simulink model "ControladoresPIDv5"  (R2020a)
settings: Solver=ode5  StartTime=0.0  StopTime=20  FixedStep=0.0001  RelTol=1e-3
values from neighbouring files (symbols this model uses):
  Bm = 0.008    [definirParametros.m]    (also in definirParametrosMotorElectroCraftDP300.m; definirParametrosMotorElectroCraftDPP728V120.m = Jm/tm; definirParametrosMotorElectroCraftDPP728V120_Optimizador.m = Jm/tm; definirParametrosMotorElectroCraftDPP728V120_v2.m = Jm/tm)
  dm = 0.3    [definirParametros.m]    (also in definirParametrosMotorElectroCraftDP300.m; definirParametrosMotorElectroCraftDPP728V120.m; definirParametrosMotorElectroCraftDPP728V120_Optimizador.m = 0.550061; definirParametrosMotorElectroCraftDPP728V120_v2.m = 0.550061)
  dmc = 0.5    [definirParametros.m]    (also in definirParametrosMotorElectroCraftDP300.m; definirParametrosMotorElectroCraftDPP728V120.m; definirParametrosMotorElectroCraftDPP728V120_Optimizador.m = 1.06911; definirParametrosMotorElectroCraftDPP728V120_v2.m = 1.06911)
  g = 9.8    [definirParametros.m]    (also in definirParametrosMotorElectroCraftDP300.m; definirParametrosMotorElectroCraftDPP728V120.m; definirParametrosMotorElectroCraftDPP728V120_Optimizador.m; definirParametrosMotorElectroCraftDPP728V120_v2.m)
  Jm = gramsCM2ToKgMeters2(12358.5)    [definirParametrosMotorElectroCraftDPP728V120.m]    (also in definirParametrosMotorElectroCraftDPP728V120_Optimizador.m; definirParametrosMotorElectroCraftDPP728V120_v2.m; definirParametrosMotorElectroCraftDPP728V120_v3.m; definirParametrosMotorElectroCraftRP34M221V90.m = gramsCM2ToKgMeters2(2718.9))
  Kb = 0.6    [definirParametros.m]    (also in definirParametrosMotorElectroCraftDP300.m = VoltagePerKRPMToVoltagePerHertz(12.3); definirParametrosMotorElectroCraftDPP728V120.m = VoltagePerKRPMToVoltagePerRadS(64.9); definirParametrosMotorElectroCraftDPP728V120_Optimizador.m = VoltagePerKRPMToVoltagePerRadS(64.9); definirParametrosMotorElectroCraftDPP728V120_v2.m = VoltagePerKRPMToVoltagePerRadS(64.9))
  Kt = 0.7274    [definirParametros.m]    (also in definirParametrosMotorElectroCraftDP300.m = newtonCMToNewtonM(11.722); definirParametrosMotorElectroCraftDPP728V120.m = newtonCMToNewtonM(62); definirParametrosMotorElectroCraftDPP728V120_Optimizador.m = newtonCMToNewtonM(62); definirParametrosMotorElectroCraftDPP728V120_v2.m = newtonCMToNewtonM(62))
  Lm = 4.3/1000    (= 0.0043)    [definirParametrosMotorElectroCraftDPP728V120.m]    (also in definirParametrosMotorElectroCraftDPP728V120_Optimizador.m; definirParametrosMotorElectroCraftDPP728V120_v2.m; definirParametrosMotorElectroCraftDPP728V120_v3.m; definirParametrosMotorElectroCraftDPP728V60.m = 0.0015)
  Mc = 200    [definirParametros.m]    (also in definirParametrosMotorElectroCraftDP300.m; definirParametrosMotorElectroCraftDPP728V120.m; definirParametrosMotorElectroCraftDPP728V120_Optimizador.m = 144.6; definirParametrosMotorElectroCraftDPP728V120_v2.m = 144.6)
  Mm = 100    [definirParametros.m]    (also in definirParametrosMotorElectroCraftDP300.m; definirParametrosMotorElectroCraftDPP728V120.m; definirParametrosMotorElectroCraftDPP728V120_Optimizador.m = 18.911; definirParametrosMotorElectroCraftDPP728V120_v2.m = 18.911)
  relacionEngranajes = 100.0/1    (= 100)    [definirParametros.m]    (also in definirParametrosMotorElectroCraftDP300.m = 1; definirParametrosMotorElectroCraftDPP728V120.m; definirParametrosMotorElectroCraftDPP728V120_Optimizador.m; definirParametrosMotorElectroCraftDPP728V120_v2.m)
  Rm = 1.55    [definirParametrosMotorElectroCraftDPP728V120.m]    (also in definirParametrosMotorElectroCraftDPP728V120_Optimizador.m; definirParametrosMotorElectroCraftDPP728V120_v2.m; definirParametrosMotorElectroCraftDPP728V120_v3.m; definirParametrosMotorElectroCraftDPP728V60.m = 0.72)
libraries: simulink x13
settings Model: Creator=rghuertaspaiva  LastModifiedBy=rghuertaspaiva

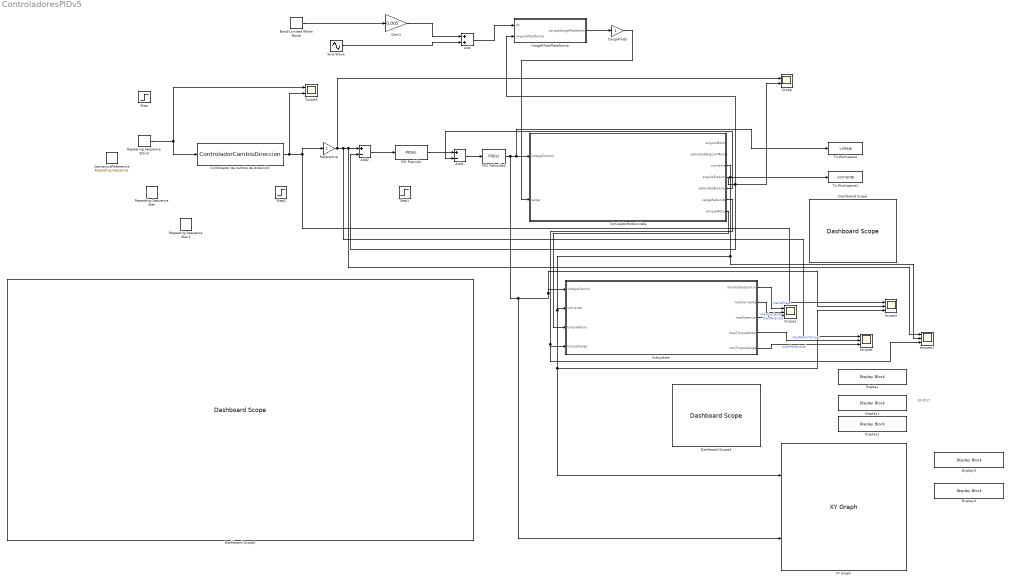
== system ControladoresPIDv5 ==
  note: 18.4917
  Add : Sum
  Add1 : Sum  Inputs=+-
  Add2 : Sum  Inputs=+-
  Band-Limited White Noise : simulink/Sources/Band-Limited White Noise  Cov=[.1]  Ts=0.001  seed=[23341]
  CargaPiloto : Gain
  CargaPilotoPlataforma : Subsystem
  Controlador de cambio de dirección : S-Function  InitFcn=try, set_param(gcb,'FunctionName','ControladorCambioDireccion'), end  FunctionName=ControladorCambioDireccion  SFunctionModules=ControladorCambioDireccion_wrapper  SFunctionDeploymentMode=off  EnableBusSupport=off  mask(S-Function Builder){}
      mask help: Simulink:masks:SFunctionBuilder_MD
      mask init:
      | val = [[.9  0.75 0.75 1 1 .9 .9 1]',[1 1 0.75 0.75 .9 .9 1 .9]'];try , sys = get_param(gcb,'SfunBuilderFcnName');if isempty(sys), sys = get_param(gcb,'FunctionName'); end,catch, sys = get_param(gcb,'FunctionName'); end
      settings: CopyFcn=set_param(gcbh,'LinkStatus','none')  PreSaveFcn=try, set_param(gcb,'FunctionName','ControladorCambioDireccion'), end  OpenFcn=sfunctionwizard(gcbh)
      mask Display: plot(val(:,1),val(:,2)),disp(sys), port_label('input',1,'entrada'), port_label('output',1,'salida')
  Dashboard Scope : DashboardScope
  Dashboard Scope2 : DashboardScope
  Dashboard Scope3 : DashboardScope
  Display{,1..4} (5 alike) : DisplayBlock  LabelPosition=Hide  Format=short  Transparency=1
  Gain1 : Gain  Gain=0.005
  PID Posiciǿn : simulink/Continuous/PID Controller  Controller=PID  Form=Parallel  TimeDomain=Continuous-time  UseExternalTs=off  SampleTime=-1  IntegratorMethod=Forward Euler  FilterMethod=Forward Euler  ControllerParametersSource=internal  P=21  I=0  D=0  UseFilter=on  N=83.8286578398202  TunerSelectOption=Transfer Function Based (PID Tuner App)  InitialConditionSource=internal  InitialConditionForIntegrator=0  InitialConditionForFilter=0  DifferentiatorICPrevScaledInput=0  ExternalReset=none  TrackingMode=off  Kt=1  LimitOutput=off  UpperSaturationLimit=inf  LowerSaturationLimit=-inf  LinearizeAsGain=on  AntiWindupMode=none  Kb=1  POutMin=[]  POutMax=[]  IOutMin=[]  IOutMax=[]  DOutMin=[]  DOutMax=[]  NOutMin=[]  NOutMax=[]  SumOutMin=[]  SumOutMax=[]  SaturationOutMin=[]  SaturationOutMax=[]  PParamMin=[]  PParamMax=[]  IParamMin=[]  IParamMax=[]  DParamMin=[]  DParamMax=[]  NParamMin=[]  NParamMax=[]  KbParamMin=[]  KbParamMax=[]  KtParamMin=[]  KtParamMax=[]  KbOutMin=[]  KbOutMax=[]  KtOutMin=[]  KtOutMax=[]  IntegratorOutMin=[]  IntegratorOutMax=[]  FilterOutMin=[]  FilterOutMax=[]  SumI1OutMin=[]  SumI1OutMax=[]  SumI2OutMin=[]  SumI2OutMax=[]  SumI3OutMin=[]  SumI3OutMax=[]  SumI4OutMin=[]  SumI4OutMax=[]  SumDOutMin=[]  SumDOutMax=[]  DifferentiatorOutMin=[]  DifferentiatorOutMax=[]  FilterDiffOutCoefMin=[]  FilterDiffOutCoefMax=[]  ReciprocalOutMin=[]  ReciprocalOutMax=[]  SumDenOutMin=[]  SumDenOutMax=[]  SumNumOutMin=[]  SumNumOutMax=[]  DivideOutMin=[]  DivideOutMax=[]  UdiffTsProdOutMin=[]  UdiffTsProdOutMax=[]  NTsProdOutMin=[]  NTsProdOutMax=[]  UintegralTsProdOutMin=[]  UintegralTsProdOutMax=[]  UngainTsProdOutMin=[]  UngainTsProdOutMax=[]  IntegratorContinuousStateAttributes=''  IntegratorStateMustResolveToSignalObject=off  IntegratorRTWStateStorageClass=Auto  FilterContinuousStateAttributes=''  FilterStateMustResolveToSignalObject=off  FilterRTWStateStorageClass=Auto  ParallelPVariant=InternalParameters  IdealPVariant=Disabled  IVariant=InternalParameters  DVariant=InternalParameters  IntegratorVariant=Continuous  SatVariant=Disabled  AWVariant=Passthrough  PCopyVariant=Disabled  TRVariant=Disabled  FdbkBlocksVariant=Forward  IdealPFdbkVariant=Disabled  SatFdbkVariant=Disabled  DerivativeFilterVariant=ContFilter  NVariant=InternalParameters  NCopyVariant=Disabled  FilterICVariant=InternalICsFilter  IntegratorICVariant=InternalICs  ExternalResetVariant=Disabled  TRSumVariant=Passthrough  SumFdbkVariant=Disabled  SumVariant=Sum_PID  TsampFilterVariant=InternalTs  TsampNgainVariant=Passthrough  TsampIntegralVariant=Passthrough
  PID Velocidad : simulink/Continuous/PID Controller  Controller=PID  Form=Parallel  TimeDomain=Continuous-time  UseExternalTs=off  SampleTime=-1  IntegratorMethod=Forward Euler  FilterMethod=Forward Euler  ControllerParametersSource=internal  P=0  I=12200  D=0  UseFilter=on  N=100  TunerSelectOption=Transfer Function Based (PID Tuner App)  InitialConditionSource=internal  InitialConditionForIntegrator=0  InitialConditionForFilter=0  DifferentiatorICPrevScaledInput=0  ExternalReset=none  TrackingMode=off  Kt=1  LimitOutput=off  UpperSaturationLimit=inf  LowerSaturationLimit=-inf  LinearizeAsGain=on  AntiWindupMode=none  Kb=1  POutMin=[]  POutMax=[]  IOutMin=[]  IOutMax=[]  DOutMin=[]  DOutMax=[]  NOutMin=[]  NOutMax=[]  SumOutMin=[]  SumOutMax=[]  SaturationOutMin=[]  SaturationOutMax=[]  PParamMin=[]  PParamMax=[]  IParamMin=[]  IParamMax=[]  DParamMin=[]  DParamMax=[]  NParamMin=[]  NParamMax=[]  KbParamMin=[]  KbParamMax=[]  KtParamMin=[]  KtParamMax=[]  KbOutMin=[]  KbOutMax=[]  KtOutMin=[]  KtOutMax=[]  IntegratorOutMin=[]  IntegratorOutMax=[]  FilterOutMin=[]  FilterOutMax=[]  SumI1OutMin=[]  SumI1OutMax=[]  SumI2OutMin=[]  SumI2OutMax=[]  SumI3OutMin=[]  SumI3OutMax=[]  SumI4OutMin=[]  SumI4OutMax=[]  SumDOutMin=[]  SumDOutMax=[]  DifferentiatorOutMin=[]  DifferentiatorOutMax=[]  FilterDiffOutCoefMin=[]  FilterDiffOutCoefMax=[]  ReciprocalOutMin=[]  ReciprocalOutMax=[]  SumDenOutMin=[]  SumDenOutMax=[]  SumNumOutMin=[]  SumNumOutMax=[]  DivideOutMin=[]  DivideOutMax=[]  UdiffTsProdOutMin=[]  UdiffTsProdOutMax=[]  NTsProdOutMin=[]  NTsProdOutMax=[]  UintegralTsProdOutMin=[]  UintegralTsProdOutMax=[]  UngainTsProdOutMin=[]  UngainTsProdOutMax=[]  IntegratorContinuousStateAttributes=''  IntegratorStateMustResolveToSignalObject=off  IntegratorRTWStateStorageClass=Auto  FilterContinuousStateAttributes=''  FilterStateMustResolveToSignalObject=off  FilterRTWStateStorageClass=Auto  ParallelPVariant=InternalParameters  IdealPVariant=Disabled  IVariant=InternalParameters  DVariant=InternalParameters  IntegratorVariant=Continuous  SatVariant=Disabled  AWVariant=Passthrough  PCopyVariant=Disabled  TRVariant=Disabled  FdbkBlocksVariant=Forward  IdealPFdbkVariant=Disabled  SatFdbkVariant=Disabled  DerivativeFilterVariant=ContFilter  NVariant=InternalParameters  NCopyVariant=Disabled  FilterICVariant=InternalICsFilter  IntegratorICVariant=InternalICs  ExternalResetVariant=Disabled  TRSumVariant=Passthrough  SumFdbkVariant=Disabled  SumVariant=Sum_PID  TsampFilterVariant=InternalTs  TsampNgainVariant=Passthrough  TsampIntegralVariant=Passthrough
  Referencia : Gain
  Repeating Sequence Stair : simulink/Sources/Repeating Sequence Stair  OutValues="[0 1 1 0 0 -1 -1  0 0  1 1 -1 -1 1 1]"  tsamp=1  OutMin=[]  OutMax=[]  OutDataTypeStr=double  OutputDataTypeScalingMode=double  OutDataType=fixdt(0,8)  ConRadixGroup=Best Precision: Vector-wise  OutScaling=2^-12
  Repeating Sequence Stair1 : simulink/Sources/Repeating Sequence Stair  OutValues="[0 1 -1 1 -1 1  -1 ]"  tsamp=1  OutMin=[]  OutMax=[]  OutDataTypeStr=double  OutputDataTypeScalingMode=double  OutDataType=fixdt(0,8)  ConRadixGroup=Best Precision: Vector-wise  OutScaling=2^-12
  Repeating Sequence Stair2 : simulink/Sources/Repeating Sequence Stair  OutValues="[0 1 1 -1 -1 1 1  -1 -1 ]"  tsamp=1  OutMin=[]  OutMax=[]  OutDataTypeStr=double  OutputDataTypeScalingMode=double  OutDataType=fixdt(0,8)  ConRadixGroup=Best Precision: Vector-wise  OutScaling=2^-12
  Scope : Scope  NumInputPorts=2
  Scope1 : Scope  NumInputPorts=3
  Scope2 : Scope  NumInputPorts=3
  Scope3 : Scope  NumInputPorts=2
  SecuenciaReferencia : simulink/Sources/Repeating Sequence  rep_seq_t=secuencia_tiempo  rep_seq_y=secuencia_valores
  SimuladorMotocicleta : Subsystem
  Sine Wave : Sin  Amplitude=0.015  Frequency=2*pi  SampleTime=0
  Step : Step  After=deg2rad(7)  SampleTime=0
  Step1 : Step  After=deg2rad(30)  SampleTime=0
  Step2 : Step  After=deg2rad(30)  SampleTime=0
  Subsystem : Subsystem
  To Workspace : ToWorkspace  VariableName=voltaje  SaveFormat=Timeseries  SampleTime=-1
  To Workspace1 : ToWorkspace  VariableName=corriente  SaveFormat=Timeseries  SampleTime=-1
  XY Graph : simulink/Sinks/XY Graph  xmin=-50  xmax=50  ymin=-80  ymax=80  st=-1
  torques : Scope  NumInputPorts=3
  torques1 : Scope  NumInputPorts=3
  wires:
  CargaPiloto/1 -> SimuladorMotocicleta/2(carga)
  Gain1/1 -> Add/1
  Sine Wave/1 -> Add/2
  Add/1 -> CargaPilotoPlataforma/1(dc)
  SimuladorMotocicleta/4(anguloExterior) -> CargaPilotoPlataforma/2(anguloPlataforma), Add2/2, Scope/2
  CargaPilotoPlataforma/1(torqueCargaPlataforma) -> CargaPiloto/1
  Band-Limited White Noise/1 -> Gain1/1
  PID Velocidad/1 -> XY Graph/2, Scope2/2, Subsystem/1(voltajeControl), To Workspace/1, SimuladorMotocicleta/1(voltajeControl)
  Add1/1 -> PID Velocidad/1
  SimuladorMotocicleta/5(velocidadExterior) -> Add1/2
  Referencia/1 -> Scope/1, torques/1, torques1/1, Add2/1
  Add2/1 -> PID Posiciǿn/1
  SimuladorMotocicleta/3(corriente) -> To Workspace1/1, torques1/2, XY Graph/1, Scope2/3, Subsystem/2(corriente)
  Subsystem/1(maxVoltajeControl) -> Scope1/1  "maxVoltaje"
  Subsystem/2(maxCorriente) -> Scope1/2  "maxCorriente"
  PID Posiciǿn/1 -> Add1/1
  Subsystem/3(maxPotencia) -> Scope1/3  "maxPotencia"
  Repeating Sequence Stair2/1 -> Controlador de cambio de dirección/1, Scope3/1
  Controlador de cambio de dirección/1 -> Scope2/1, Referencia/1, Scope3/2
  Subsystem/4(maxTorqueMotor) -> torques/2  "maxMotorTorque"
  Subsystem/5(maxTorqueCarga) -> torques/3  "maxMeterLoad"
  SimuladorMotocicleta/7(torqueMotor) -> Subsystem/3(torqueMotor)
  SimuladorMotocicleta/6(cargaReducida) -> torques1/3, Subsystem/4(torqueCarga)

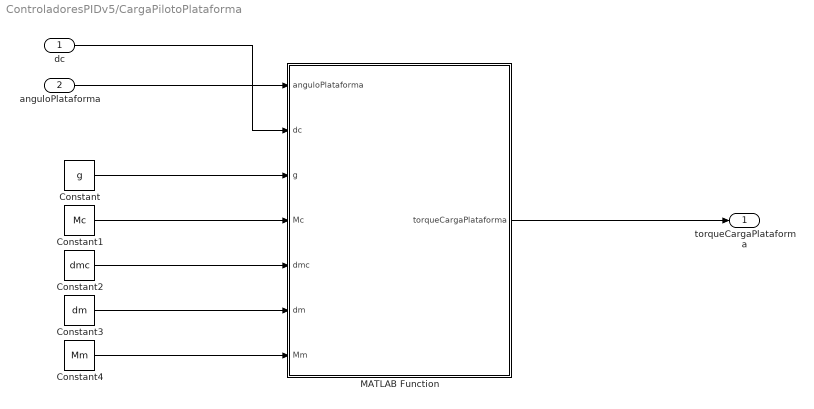
== system ControladoresPIDv5/CargaPilotoPlataforma ==
  dc : Inport
  anguloPlataforma : Inport  Port=2
  Constant : Constant  Value=g
  Constant1 : Constant  Value=Mc
  Constant2 : Constant  Value=dmc
  Constant3 : Constant  Value=dm
  Constant4 : Constant  Value=Mm
  MATLAB Function : MATLAB Function  TreatAsAtomicUnit=on
  torqueCargaPlataforma : Outport
  wires:
  dc/1 -> MATLAB Function/2(dc)
  anguloPlataforma/1 -> MATLAB Function/1(anguloPlataforma)
  Constant/1 -> MATLAB Function/3(g)
  Constant1/1 -> MATLAB Function/4(Mc)
  Constant2/1 -> MATLAB Function/5(dmc)
  Constant3/1 -> MATLAB Function/6(dm)
  Constant4/1 -> MATLAB Function/7(Mm)
  MATLAB Function/1(torqueCargaPlataforma) -> torqueCargaPlataforma/1

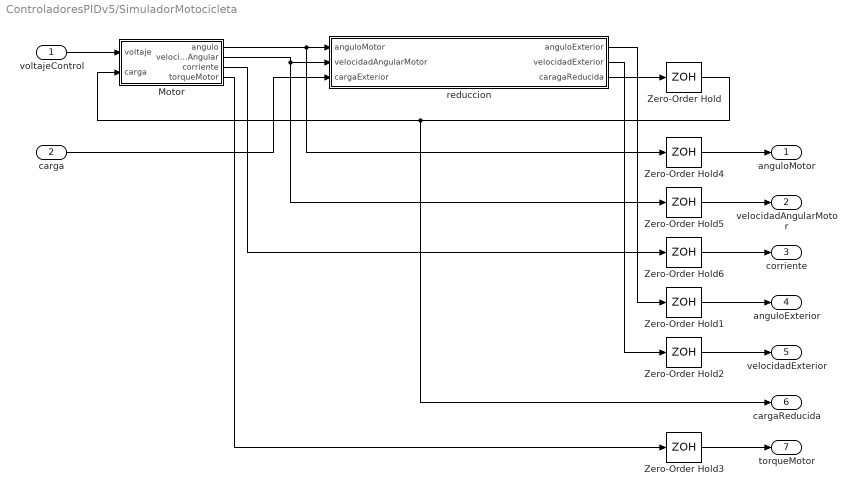
== system ControladoresPIDv5/SimuladorMotocicleta ==
  voltajeControl : Inport
  carga : Inport  Port=2
  Motor : Subsystem
  Zero-Order Hold{,1..6} (7 alike) : ZeroOrderHold  SampleTime=-1
  reduccion : Subsystem
  anguloMotor : Outport
  velocidadAngularMotor : Outport  Port=2
  corriente : Outport  Port=3
  anguloExterior : Outport  Port=4
  velocidadExterior : Outport  Port=5
  cargaReducida : Outport  Port=6
  torqueMotor : Outport  Port=7
  wires:
  voltajeControl/1 -> Motor/1(voltaje)
  Motor/1(angulo) -> Zero-Order Hold4/1, reduccion/1(anguloMotor)
  Motor/2(velocidadAngular) -> Zero-Order Hold5/1, reduccion/2(velocidadAngularMotor)
  carga/1 -> reduccion/3(cargaExterior)
  reduccion/3(caragaReducida) -> Zero-Order Hold/1
  Motor/3(corriente) -> Zero-Order Hold6/1
  reduccion/1(anguloExterior) -> Zero-Order Hold1/1
  reduccion/2(velocidadExterior) -> Zero-Order Hold2/1
  Zero-Order Hold1/1 -> anguloExterior/1
  Zero-Order Hold2/1 -> velocidadExterior/1
  Zero-Order Hold/1 -> cargaReducida/1, Motor/2(carga)
  Zero-Order Hold4/1 -> anguloMotor/1
  Zero-Order Hold5/1 -> velocidadAngularMotor/1
  Zero-Order Hold6/1 -> corriente/1
  Motor/4(torqueMotor) -> Zero-Order Hold3/1
  Zero-Order Hold3/1 -> torqueMotor/1

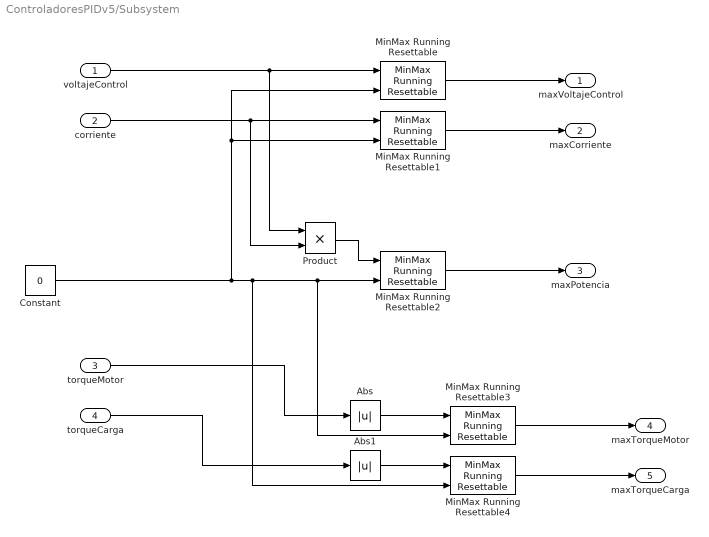
== system ControladoresPIDv5/Subsystem ==
  voltajeControl : Inport
  corriente : Inport  Port=2
  torqueMotor : Inport  Port=3
  torqueCarga : Inport  Port=4
  Abs : Abs
  Abs1 : Abs
  Constant : Constant  Value=0
  MinMax Running Resettable{,1..4} (5 alike) : simulink/Math Operations/MinMax Running Resettable  Function=max  vinit=0.0
  Product : Product
  maxVoltajeControl : Outport
  maxCorriente : Outport  Port=2
  maxPotencia : Outport  Port=3
  maxTorqueMotor : Outport  Port=4
  maxTorqueCarga : Outport  Port=5
  wires:
  voltajeControl/1 -> Product/1, MinMax Running Resettable/1
  corriente/1 -> Product/2, MinMax Running Resettable1/1
  Constant/1 -> MinMax Running Resettable1/2, MinMax Running Resettable/2, MinMax Running Resettable4/2, MinMax Running Resettable3/2, MinMax Running Resettable2/2
  MinMax Running Resettable/1 -> maxVoltajeControl/1
  MinMax Running Resettable1/1 -> maxCorriente/1
  Product/1 -> MinMax Running Resettable2/1
  MinMax Running Resettable2/1 -> maxPotencia/1
  MinMax Running Resettable4/1 -> maxTorqueCarga/1
  MinMax Running Resettable3/1 -> maxTorqueMotor/1
  torqueMotor/1 -> Abs/1
  torqueCarga/1 -> Abs1/1
  Abs/1 -> MinMax Running Resettable3/1
  Abs1/1 -> MinMax Running Resettable4/1

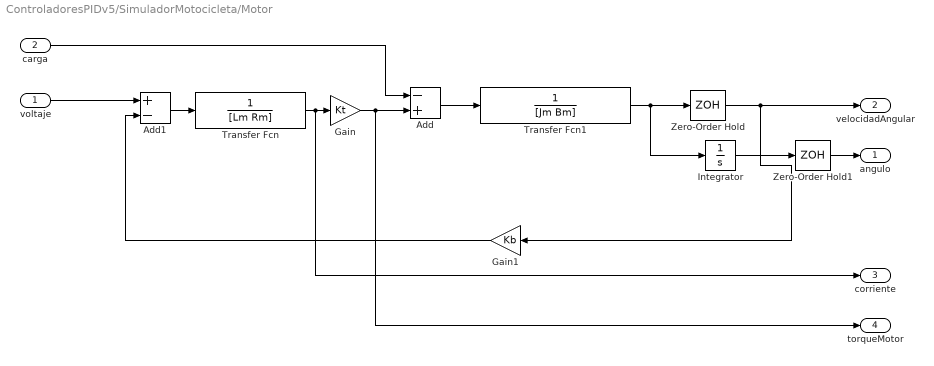
== system ControladoresPIDv5/SimuladorMotocicleta/Motor ==
  voltaje : Inport
  carga : Inport  Port=2
  Add : Sum  Inputs=-+
  Add1 : Sum  Inputs=+-
  Gain : Gain  Gain=Kt
  Gain1 : Gain  Gain=Kb
  Integrator : Integrator
  Transfer Fcn : TransferFcn  Denominator=[Lm Rm]
  Transfer Fcn1 : TransferFcn  Denominator=[Jm Bm]
  Zero-Order Hold : ZeroOrderHold  SampleTime=-1
  Zero-Order Hold1 : ZeroOrderHold  SampleTime=-1
  angulo : Outport
  velocidadAngular : Outport  Port=2
  corriente : Outport  Port=3
  torqueMotor : Outport  Port=4
  wires:
  Gain/1 -> torqueMotor/1, Add/2
  Add/1 -> Transfer Fcn1/1
  Transfer Fcn/1 -> corriente/1, Gain/1
  Transfer Fcn1/1 -> Integrator/1, Zero-Order Hold/1
  Zero-Order Hold/1 -> Gain1/1, velocidadAngular/1
  Integrator/1 -> Zero-Order Hold1/1
  voltaje/1 -> Add1/1
  Add1/1 -> Transfer Fcn/1
  Gain1/1 -> Add1/2
  carga/1 -> Add/1
  Zero-Order Hold1/1 -> angulo/1

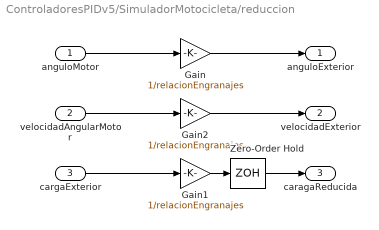
== system ControladoresPIDv5/SimuladorMotocicleta/reduccion ==
  anguloMotor : Inport
  velocidadAngularMotor : Inport  Port=2
  cargaExterior : Inport  Port=3
  Gain : Gain  Gain=1/relacionEngranajes
  Gain1 : Gain  Gain=1/relacionEngranajes
  Gain2 : Gain  Gain=1/relacionEngranajes
  Zero-Order Hold : ZeroOrderHold  SampleTime=-1
  anguloExterior : Outport
  velocidadExterior : Outport  Port=2
  caragaReducida : Outport  Port=3
  wires:
  anguloMotor/1 -> Gain/1
  Gain/1 -> anguloExterior/1
  cargaExterior/1 -> Gain1/1
  Gain1/1 -> Zero-Order Hold/1
  velocidadAngularMotor/1 -> Gain2/1
  Gain2/1 -> velocidadExterior/1
  Zero-Order Hold/1 -> caragaReducida/1

== matlab function ControladoresPIDv5/CargaPilotoPlataforma/MATLAB Function ==
  data: anguloPlataforma input; torqueCargaPlataforma output; dc input; g input; Mc input; dmc input; dm input; Mm input
function torqueCargaPlataforma = torquePlataformaPiloto(anguloPlataforma, dc, g, Mc, dmc, dm, Mm)

%torqueCargaPlataforma = 0;
% torqueCargaPlataforma = g*( dc*Mc*cos(anguloPlataforma) + ...
%                             (dmc*Mc + dm*(Mc + Mm))*sin(anguloPlataforma) ...
%                           );
torqueCargaPlataforma =  g*( 0*Mc*cos(anguloPlataforma) + ...
                             (dmc*Mc + dm*(Mc + Mm))*sin(anguloPlataforma) ...
                           );
%t=0;
